simulink library "HX_tube_stratified"  (R2016b)
settings: Solver=ode45  StartTime=0.0  StopTime=10.0  RelTol=1e-3  EnableMultiTasking=on
libraries: carnot x2
settings Model: Creator=lena.frank  LastModifiedBy=drhf
settings DataIOCC: LimitDataPoints=on  SaveFormat=Array  SignalLoggingSaveFormat=ModelDataLogs
settings OptimizationCC: ExpressionDepthLimit=2147483647  LifeSpan=inf
settings DebuggingCC: UnderspecifiedInitializationDetection=Classic  MergeDetectMultiDrivingBlocksExec=none  SolverPrmCheckMsg=warning  FcnCallInpInsideContextMsg=warning  StateNameClashWarn=warning  SFUnexpectedBacktrackingDiag=warning  SFNoUnconditionalDefaultTransitionDiag=warning  SFExecutionAtInitializationDiag=none
settings HardwareCC: ProdBitPerPointer=32  ProdBitPerSizeT=32  ProdBitPerPtrDiffT=32  ProdLargestAtomicFloat=None  ProdIntDivRoundTo=Undefined  ProdEndianess=Unspecified  ProdWordSize=32  ProdHWDeviceType=32-bit Generic
settings ModelReferenceCC: PropagateSignalLabelsOutOfModel=off
settings GRTTargetCC: TargetLangStandard=C89/C90 (ANSI)  GeneratePreprocessorConditionals=Disable all  CombineOutputUpdateFcns=off  GRTInterface=on
settings ConfigComp: CovMetricSettings=dw  CovHtmlReporting=on  CovSaveCumulativeToWorkspaceVar=on  CovSaveSingleToWorkspaceVar=on  CovExternalEMLEnable=off

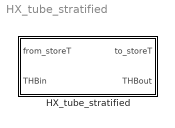
== system HX_tube_stratified ==
  HX_tube_stratified : Subsystem  mask(smooth tube heat exchanger for storage){h_in=1, h_out=0, hgt=1.5, dpipe=0.03, swall=0.001, lpipe=10, cond=50, height=-1.5, dplin=100, dpqua=100, nodes=10}
      mask prompts: h_in "relative height of inlet"; h_out "relative height of outlet"; hgt "Height of storage in m"; dpipe "outer diameter of HX pipe in m"; swall "thickness of pipe wall in m"; lpipe "length of HX pipe in m"; cond "thermal conductivity of HX wall in W/m/K"; height "Height difference inlet-outlet [m]"; dplin "Pressure drop coefficient dplin [Pa/(kg/s)]"; dpqua "Pressure drop coefficient dpqua [Pa/(kg/s)²]"; nodes "number of nodes"
      mask help:
      | The block transforms the incoming THV vector to a vector which the storage interprets as a heat exchanger.
      | Give inlet and outlet as a relative position 0=bottom to 1=top
      | The heat transfer is calculated with an equation from Wagner: Waermeuebertragung, Vogel-Verlag, 1991
      mask init:
      | in = zeros(nodes,1);    % vector of length nodes
      | up = in;                % vector of length nodes
      | down = in;              % vector of length nodes
      | 
      | h_in = max(0,h_in);     % no nodes below 0
      | h_out = max(0,h_out);   % no nodes below 0
      | 
      | inlet = round(h_in*(nodes-1))+1;    % inlet position
      | outlet = round(h_out*(nodes-1))+1;  % outlet position
      | set_param(gcb,'height',num2str((h_out-h_in)*hgt));
      | % hgt = (h_out-h_in)*hgt;
      | 
      | in(inlet)=1;
      | 
      | if (h_in < h_out)           % if inlet below outlet
      |     up(inlet:outlet)=1;     % upwards
      | elseif (h_in > h_out)       % else if inlet above outlet
      |     down(outlet:inlet)=1;   % downwards
      | end
      mask Help: web(['file:///' fullfile(path_carnot('help'),'StoragePorts_HeatExchangerModels.html')],'-helpbrowser')
      mask TypeOptions dpipe: sfun_storage_heatexchanger/p1
      mask TypeOptions swall: sfun_storage_heatexchanger/p2
      mask TypeOptions lpipe: sfun_storage_heatexchanger/p3
      mask TypeOptions cond: sfun_storage_heatexchanger/p4
      mask TypeOptions height: Pressure_Drop_StorageHX/hgt
      mask TypeOptions dplin: Pressure_Drop_StorageHX/dplin
      mask TypeOptions dpqua: Pressure_Drop_StorageHX/dpqua
      mask TypeOptions nodes: sfun_storage_heatexchanger/nodes
      mask Display: disp('HX tube STRAT')

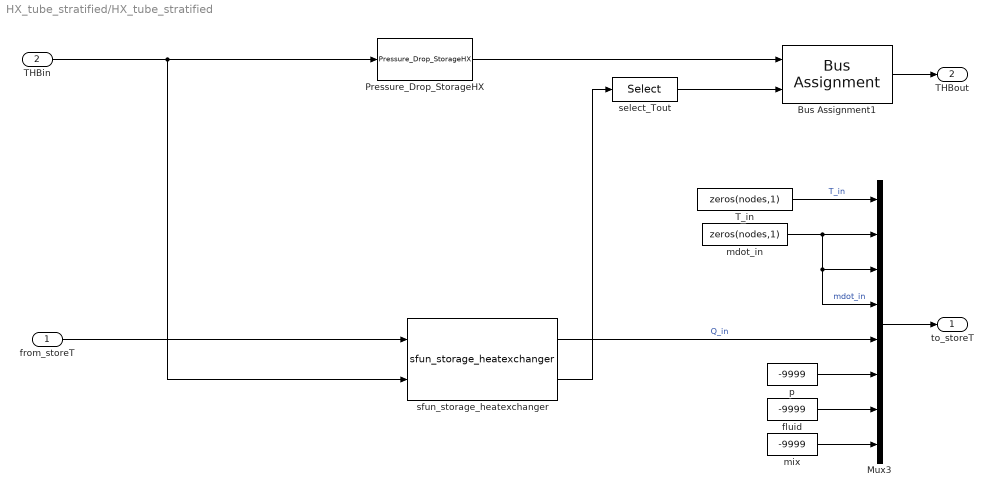
== system HX_tube_stratified/HX_tube_stratified ==
  from_storeT : Inport
  THBin : Inport  Port=2
  Bus Assignment1 : BusAssignment  AssignedSignals=Temperature
  Mux3 : Mux  Inputs=8
  Pressure_Drop_StorageHX : carnot/Basic/Pressure_Drop/Pressure_Drop_StorageHX  dia=dia  hgt=height  dplin=dplin  dpqua=dpqua
  T_in : Constant  Value=zeros(nodes,1)
  fluid : Constant  Value=-9999
  mdot_in : Constant  Value=zeros(nodes,1)
  mix : Constant  Value=-9999
  p : Constant  Value=-9999
  select_Tout : Selector  InputPortWidth=nodes  IndexOptions=Index vector (dialog)  Indices=[outlet]  OutputSizes=1
  sfun_storage_heatexchanger : carnot/Basic/Thermal_Models/sfun_storage_heatexchanger  idn=smooth tube theoretical - stratified  nodes=nodes  inlet=inlet  outlet=outlet  p1=dpipe  p2=swall  p3=lpipe  p4=cond  p5=0  p6=0  p7=0
  to_storeT : Outport
  THBout : Outport  Port=2
  wires:
  Pressure_Drop_StorageHX/1 -> Bus Assignment1/1
  sfun_storage_heatexchanger/2 -> select_Tout/1
  mix/1 -> Mux3/8
  fluid/1 -> Mux3/7
  p/1 -> Mux3/6
  Bus Assignment1/1 -> THBout/1
  sfun_storage_heatexchanger/1 -> Mux3/5  "Q_in"
  T_in/1 -> Mux3/1  "T_in"
  select_Tout/1 -> Bus Assignment1/2
  Mux3/1 -> to_storeT/1
  mdot_in/1 -> Mux3/4, Mux3/3, Mux3/2  "mdot_in"
  THBin/1 -> Pressure_Drop_StorageHX/1, sfun_storage_heatexchanger/2
  from_storeT/1 -> sfun_storage_heatexchanger/1
